simulink model "error_tracker"  (R2025b)
settings: Solver=VariableStepAuto  StartTime=0.0  StopTime=10.0  RelTol=1e-3
settings Model: Creator=samue  LastModifiedBy=samue

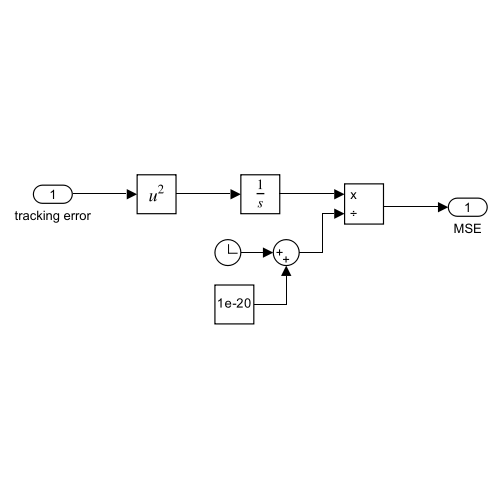
[thumbnail: Simulink's stored preview of the top-level diagram]
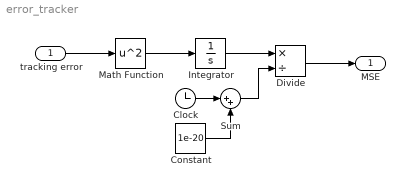
== system error_tracker ==
  tracking error : Inport
  Clock : Clock
  Constant : Constant  Value=1e-20
  Divide : Product  Inputs=*/
  Integrator : Integrator
  Math Function : Math  Operator=square
  Sum : Sum  Inputs=|++
  MSE : Outport
  wires:
  Integrator/1 -> Divide/1
  Math Function/1 -> Integrator/1
  Clock/1 -> Sum/1
  Divide/1 -> MSE/1
  Sum/1 -> Divide/2
  Constant/1 -> Sum/2
  tracking error/1 -> Math Function/1
